simulink model "barra1"  (R2018a)
settings: Solver=ode45  StartTime=0.0  StopTime=tfinal  RelTol=1e-6  EnableMultiTasking=on
undefined symbols (not defined in the file): barrassmodel, Ts
settings Model: Creator=jomle  LastModifiedBy=leonardopedroso
settings DataIOCC: LimitDataPoints=on  SaveFormat=Array
settings OptimizationCC: LifeSpan=inf
settings DebuggingCC: SFUnexpectedBacktrackingDiag=warning  SFNoUnconditionalDefaultTransitionDiag=warning  SFExecutionAtInitializationDiag=none
settings HardwareCC: ProdBitPerPointer=32  ProdBitPerSizeT=32  ProdBitPerPtrDiffT=32  ProdLargestAtomicFloat=None  ProdIntDivRoundTo=Undefined  ProdEndianess=Unspecified  ProdWordSize=32  ProdHWDeviceType=32-bit Generic
settings ModelReferenceCC: PropagateSignalLabelsOutOfModel=off
settings CodeAppCC: StateflowObjectComments=on
settings GRTTargetCC: TargetLangStandard=C89/C90 (ANSI)  GeneratePreprocessorConditionals=Disable all
settings ConfigComp: CovMetricSettings=dw  CovHtmlReporting=on  CovSaveCumulativeToWorkspaceVar=on  CovSaveSingleToWorkspaceVar=on  CovExternalEMLEnable=off

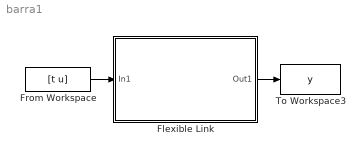
== system barra1 ==
  Flexible Link : Subsystem
      mask Display: image('./model/quanserlink.jpg');
  From Workspace : FromWorkspace  VariableName=[t u]  SampleTime=0  Interpolate=off  OutputAfterFinalValue=Setting to zero
  To Workspace3 : ToWorkspace  VariableName=y  SampleTime=Ts
  wires:
  From Workspace/1 -> Flexible Link/1(In1)
  Flexible Link/1(Out1) -> To Workspace3/1

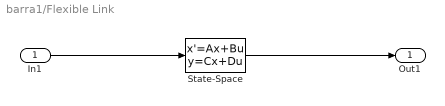
== system barra1/Flexible Link ==
  In1 : Inport
  State-Space : StateSpace  A=barrassmodel.Atrue  B=barrassmodel.Btrue  C=barrassmodel.Ctrue  D=barrassmodel.Dtrue  InitialCondition=0
  Out1 : Outport
  wires:
  State-Space/1 -> Out1/1
  In1/1 -> State-Space/1
